simulink model "slb_name"  (R2015b)
settings: Solver=FixedStepDiscrete  SolverMode=SingleTasking  StartTime=0.0  StopTime=3  RelTol=1e-3
libraries: simulink x2
settings Model: Creator=at-mt  LastModifiedBy=amatsumo
settings DataIOCC: SaveFormat=Array  SignalLoggingSaveFormat=ModelDataLogs  SaveOutput=off  SignalLogging=off  SaveTime=off
settings OptimizationCC: BlockReduction=off  ConditionallyExecuteInputs=off  DefaultParameterBehavior=Inlined  ExpressionDepthLimit=2147483647
settings DebuggingCC: AlgebraicLoopMsg=error  UnderspecifiedInitializationDetection=Classic  MergeDetectMultiDrivingBlocksExec=none  SolverPrmCheckMsg=warning  SingleTaskRateTransMsg=error  FcnCallInpInsideContextMsg=UseLocalSettings  StateNameClashWarn=warning
settings HardwareCC: ProdBitPerPointer=32  ProdLargestAtomicFloat=None  ProdIntDivRoundTo=Undefined  ProdEndianess=Unspecified  ProdWordSize=32  ProdHWDeviceType=ASIC/FPGA->ASIC/FPGA  ProdEqTarget=off
settings SFSimCC: SFSimEcho=off  SimParseCustomCode=off
settings GRTTargetCC: GeneratePreprocessorConditionals=Disable all  CombineOutputUpdateFcns=off  GRTInterface=on
settings ConfigComp: CovModelRefEnable=Off  CovSFcnEnable=off

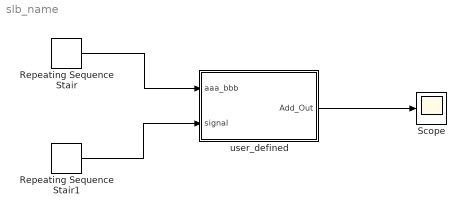
== system slb_name ==
  Repeating Sequence Stair : simulink/Sources/Repeating Sequence Stair  OutValues=[3 1 4 2 1 12 -11].'  tsamp=1  OutMin=[]  OutMax=[]  OutDataTypeStr=int8  OutputDataTypeScalingMode=int8  OutDataType=fixdt(0,8)  ConRadixGroup=Best Precision: Vector-wise  OutScaling=2^-12
  Repeating Sequence Stair1 : simulink/Sources/Repeating Sequence Stair  OutValues=[8 4 5 3 9 15 2 -4 -8].'  tsamp=1  OutMin=[]  OutMax=[]  OutDataTypeStr=int8  OutputDataTypeScalingMode=int8  OutDataType=fixdt(0,8)  ConRadixGroup=Best Precision: Vector-wise  OutScaling=2^-12
  Scope : Scope
  user_defined : Subsystem
  wires:
  Repeating Sequence Stair/1 -> user_defined/1(aaa_bbb)
  Repeating Sequence Stair1/1 -> user_defined/2(signal)
  user_defined/1(Add_Out) -> Scope/1

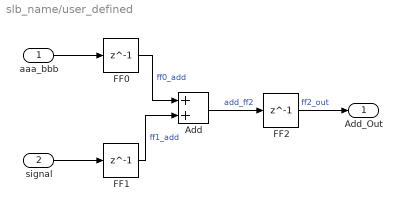
== system slb_name/user_defined ==
  aaa_bbb : Inport
  signal : Inport  Port=2
  Add : Sum
  FF0 : Delay  DelayLength=1
  FF1 : Delay  DelayLength=1
  FF2 : Delay  DelayLength=1
  Add_Out : Outport
  wires:
  FF1/1 -> Add/2  "ff1_add"
  signal/1 -> FF1/1
  Add/1 -> FF2/1  "add_ff2"
  FF2/1 -> Add_Out/1  "ff2_out"
  aaa_bbb/1 -> FF0/1
  FF0/1 -> Add/1  "ff0_add"
